simulink model "Hinf_design"  (R2019b)
settings: Solver=ode14x  StartTime=0.0  StopTime=experiment.stop_time  FixedStep=0.002  RelTol=1e-3
values from neighbouring files (symbols this model uses):
  B_1 = B    (= 0.0015)    [nominal_model.m]
  B_2 = B    (= 0.0015)    [nominal_model.m]
  B_eq = 0.015    [nominal_model.m]
  data = e_h.load_data    [potentiometer_recover.m]
  eta_g = 0.9    [nominal_model.m]
  eta_m = 0.69    [nominal_model.m]
  experiment = merge( experiment, experiment2 )    [blackbox_est.m]
  J_1 = J    (= 0.000545)    [nominal_model.m]
  J_2 = J    (= 0.000545)    [nominal_model.m]
  J_eq = 2.087e-3    (= 0.002087)    [nominal_model.m]
  K_g = 70    [nominal_model.m]
  k_m = 7.68e-3    (= 0.00768)    [nominal_model.m]
  K_s1 = K_s    (= 1)    [nominal_model.m]
  K_s2 = K_s    (= 1)    [nominal_model.m]
  k_t = 7.68e-3    (= 0.00768)    [nominal_model.m]
  Lm = 0.18e-3    (= 0.00018)    [nominal_model.m]
  Rm = 2.6    [nominal_model.m]
  V_max = 10    [nominal_model.m]
undefined symbols (not defined in the file or in its folder): active_dof, controller, encoder_var, potentiometer_var
libraries: simulink x12
settings Model: Creator=giacomo  LastModifiedBy=denniszanutto

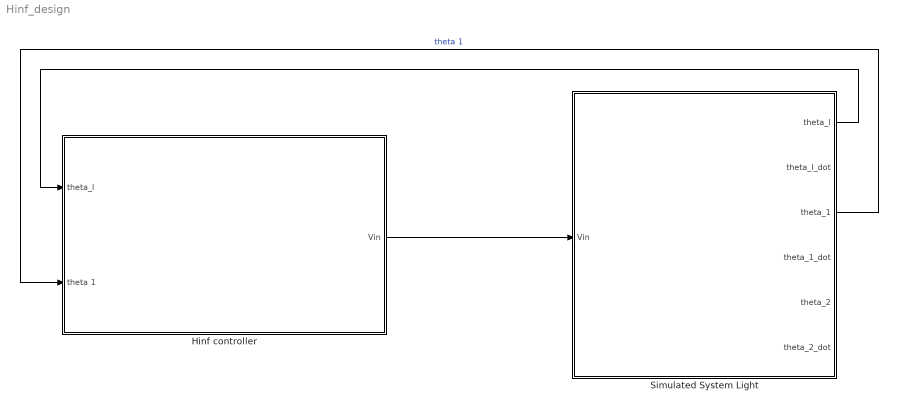
== system Hinf_design ==
  Hinf controller : Subsystem
  Simulated System Light : Subsystem
  wires:
  Simulated System Light/1(theta_l) -> Hinf controller/1(theta_l)
  Simulated System Light/3(theta_1) -> Hinf controller/2(theta 1)  "theta 1"
  Hinf controller/1(Vin) -> Simulated System Light/1(Vin)

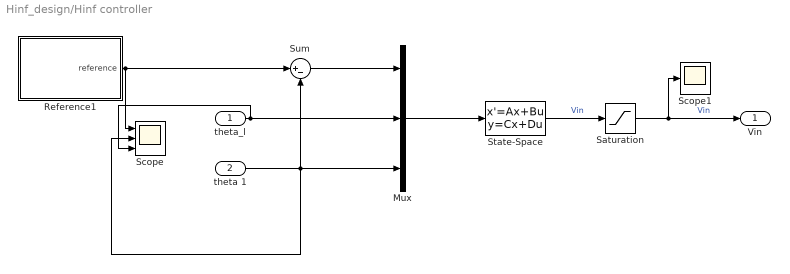
== system Hinf_design/Hinf controller ==
  theta_l : Inport
  theta 1 : Inport  Port=2
  Mux : Mux  Inputs=3
  Reference1 : Subsystem
  Saturation : Saturate  UpperLimit=V_max  LowerLimit=-V_max
  Scope : Scope  NumInputPorts=3
  Scope1 : Scope
  State-Space : StateSpace  A=controller.c11.A  B=controller.c11.B  C=controller.c11.C  D=controller.c11.D  InitialCondition=0
  Sum : Sum  Inputs=|+-
  Vin : Outport
  wires:
  Reference1/1(reference) -> Sum/1, Scope/1
  State-Space/1 -> Saturation/1  "Vin"
  Sum/1 -> Mux/1
  theta_l/1 -> Scope/3, Mux/2
  theta 1/1 -> Scope/2, Mux/3, Sum/2
  Mux/1 -> State-Space/1
  Saturation/1 -> Vin/1, Scope1/1  "Vin"

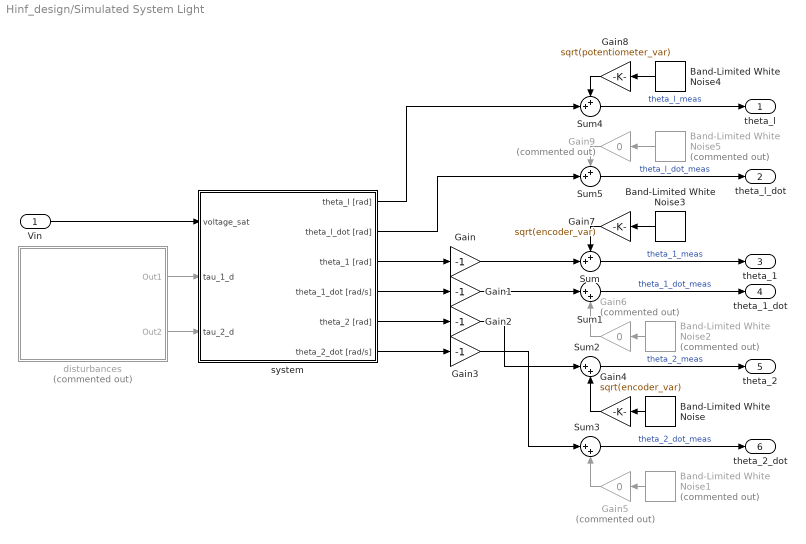
== system Hinf_design/Simulated System Light ==
  Vin : Inport
  Band-Limited White Noise : simulink/Sources/Band-Limited White Noise  Cov=1  Ts=0.002  seed=[23341]
  Band-Limited White Noise1 : simulink/Sources/Band-Limited White Noise  Commented=on  Cov=1  Ts=0.002  seed=[23341]
  Band-Limited White Noise2 : simulink/Sources/Band-Limited White Noise  Commented=on  Cov=1  Ts=0.002  seed=[23341]
  Band-Limited White Noise3 : simulink/Sources/Band-Limited White Noise  Cov=1  Ts=0.002  seed=[23341]
  Band-Limited White Noise4 : simulink/Sources/Band-Limited White Noise  Cov=1  Ts=0.002  seed=[23341]
  Band-Limited White Noise5 : simulink/Sources/Band-Limited White Noise  Commented=on  Cov=1  Ts=0.002  seed=[23341]
  Gain{,1..3} (4 alike) : Gain  Gain=-1
  Gain4 : Gain  Gain=sqrt(encoder_var)
  Gain5 : Gain  Commented=on  Gain=0
  Gain6 : Gain  Commented=on  Gain=0
  Gain7 : Gain  Gain=sqrt(encoder_var)
  Gain8 : Gain  Gain=sqrt(potentiometer_var)
  Gain9 : Gain  Commented=on  Gain=0
  Sum : Sum  Inputs=++|
  Sum1 : Sum  Inputs=|++
  Sum2 : Sum  Inputs=|++
  Sum3 : Sum  Inputs=|++
  Sum4 : Sum  Inputs=++|
  Sum5 : Sum  Inputs=++|
  disturbances : Subsystem  Commented=on
  system : Subsystem
  theta_l : Outport
  theta_l_dot : Outport  Port=2
  theta_1 : Outport  Port=3
  theta_1_dot : Outport  Port=4
  theta_2 : Outport  Port=5
  theta_2_dot : Outport  Port=6
  wires:
  system/5(theta_2 [rad]) -> Gain2/1
  system/6(theta_2_dot [rad/s]) -> Gain3/1
  system/4(theta_1_dot [rad/s]) -> Gain1/1
  Vin/1 -> system/1(voltage_sat)
  Gain/1 -> Sum/2
  Gain2/1 -> Sum2/1
  system/3(theta_1 [rad]) -> Gain/1
  Sum/1 -> theta_1/1  "theta_1_meas"
  Sum1/1 -> theta_1_dot/1  "theta_1_dot_meas"
  Sum2/1 -> theta_2/1  "theta_2_meas"
  Gain3/1 -> Sum3/1
  Sum3/1 -> theta_2_dot/1  "theta_2_dot_meas"
  Gain4/1 -> Sum2/2
  Band-Limited White Noise/1 -> Gain4/1
  Band-Limited White Noise1/1 -> Gain5/1
  Gain5/1 -> Sum3/2
  Band-Limited White Noise2/1 -> Gain6/1
  Gain7/1 -> Sum/1
  Band-Limited White Noise3/1 -> Gain7/1
  Gain8/1 -> Sum4/1
  Band-Limited White Noise4/1 -> Gain8/1
  Sum4/1 -> theta_l/1  "theta_l_meas"
  Sum5/1 -> theta_l_dot/1  "theta_l_dot_meas"
  Band-Limited White Noise5/1 -> Gain9/1
  Gain9/1 -> Sum5/1
  system/2(theta_l_dot [rad]) -> Sum5/2
  system/1(theta_l [rad]) -> Sum4/2
  Gain1/1 -> Sum1/1
  Gain6/1 -> Sum1/2
  disturbances/1(Out1) -> system/2(tau_1_d)
  disturbances/2(Out2) -> system/3(tau_2_d)

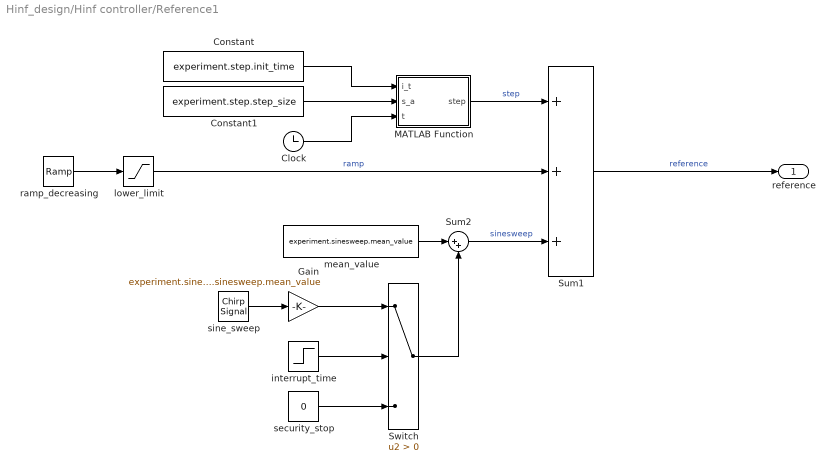
== system Hinf_design/Hinf controller/Reference1 ==
  Clock : Clock
  Constant : Constant  Value=experiment.step.init_time
  Constant1 : Constant  Value=experiment.step.step_size
  Gain : Gain  Gain=experiment.sinesweep.v_max-experiment.sinesweep.mean_value
  MATLAB Function : MATLAB Function  TreatAsAtomicUnit=on
  Sum1 : Sum  Inputs=+++
  Sum2 : Sum  Inputs=|++
  Switch : Switch  Criteria=u2 > Threshold
  interrupt_time : Step  Time=experiment.sinesweep.target_time  Before=1  After=-1  SampleTime=0
  lower_limit : Saturate  UpperLimit=max( experiment.ramp.init_value, experiment.ramp.final_value )  LowerLimit=min( experiment.ramp.init_value, experiment.ramp.final_value )
  mean_value : Constant  Value=experiment.sinesweep.mean_value
  ramp_decreasing : simulink/Sources/Ramp  slope=experiment.ramp.ramp_pend  start=experiment.ramp.init_time  InitialOutput=experiment.ramp.init_value
  security_stop : Constant  Value=0
  sine_sweep : simulink/Sources/Chirp Signal  f1=experiment.sinesweep.init_freq  T=experiment.sinesweep.target_time  f2=experiment.sinesweep.final_freq
  reference : Outport
  wires:
  mean_value/1 -> Sum2/1
  lower_limit/1 -> Sum1/2  "ramp"
  Switch/1 -> Sum2/2
  interrupt_time/1 -> Switch/2
  Sum2/1 -> Sum1/3  "sinesweep"
  Sum1/1 -> reference/1  "reference"
  security_stop/1 -> Switch/3
  ramp_decreasing/1 -> lower_limit/1
  Gain/1 -> Switch/1
  sine_sweep/1 -> Gain/1
  Clock/1 -> MATLAB Function/3(t)
  Constant/1 -> MATLAB Function/1(i_t)
  Constant1/1 -> MATLAB Function/2(s_a)
  MATLAB Function/1(step) -> Sum1/1  "step"

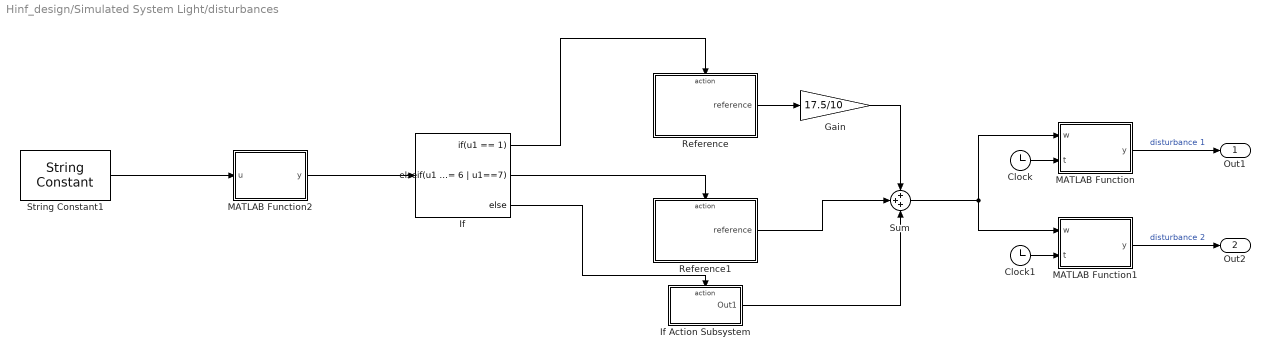
== system Hinf_design/Simulated System Light/disturbances ==
  Clock : Clock
  Clock1 : Clock
  Gain : Gain  Gain=17.5/10
  If : If  IfExpression=u1 == 1  ElseIfExpressions=u1 == 5 | u1 == 6 | u1==7
  If Action Subsystem : Subsystem  TreatAsAtomicUnit=on
  MATLAB Function : MATLAB Function  TreatAsAtomicUnit=on
  MATLAB Function1 : MATLAB Function  TreatAsAtomicUnit=on
  MATLAB Function2 : MATLAB Function  TreatAsAtomicUnit=on
  Reference : Subsystem
  Reference1 : Subsystem
  String Constant1 : StringConstant  String=experiment.refVariable
  Sum : Sum  Inputs=+++
  Out1 : Outport
  Out2 : Outport  Port=2
  wires:
  Clock/1 -> MATLAB Function/2(t)
  MATLAB Function/1(y) -> Out1/1  "disturbance 1"
  Clock1/1 -> MATLAB Function1/2(t)
  MATLAB Function1/1(y) -> Out2/1  "disturbance 2"
  Reference/1(reference) -> Gain/1
  If/1 -> Reference/Action
  MATLAB Function2/1(y) -> If/1
  If/2 -> Reference1/Action
  If/3 -> If Action Subsystem/Action
  Gain/1 -> Sum/1
  Reference1/1(reference) -> Sum/2
  If Action Subsystem/1(Out1) -> Sum/3
  Sum/1 -> MATLAB Function1/1(w), MATLAB Function/1(w)
  String Constant1/1 -> MATLAB Function2/1(u)

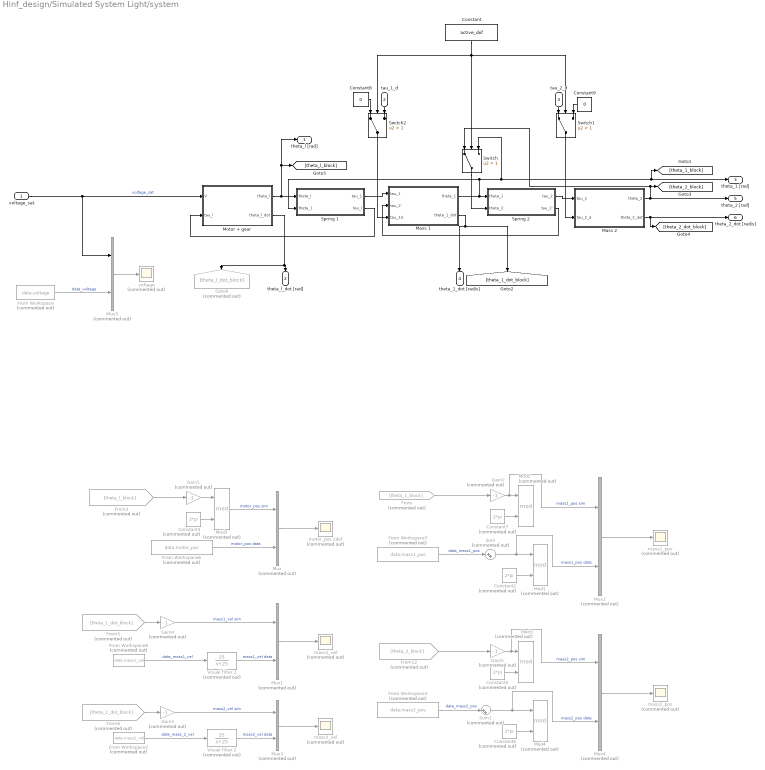
== system Hinf_design/Simulated System Light/system ==
  voltage_sat : Inport
  tau_1_d : Inport  Port=2
  tau_2_d : Inport  Port=3
  Constant : Constant  Value=active_dof
  Constant{2..4,6..7} (5 alike) : Constant  Commented=on  Value=2*pi
  Constant8 : Constant  Value=0
  Constant9 : Constant  Value=0
  From : From  Commented=on  GotoTag=theta_1_block
  From Workspace : FromWorkspace  Commented=on  VariableName=data.voltage  SampleTime=0
  From Workspace2 : FromWorkspace  Commented=on  VariableName=data.mass2_vel  SampleTime=0.002
  From Workspace3 : FromWorkspace  Commented=on  VariableName=data.mass2_pos  SampleTime=0.002
  From Workspace6 : FromWorkspace  Commented=on  VariableName=data.motor_pos  SampleTime=0.002
  From Workspace7 : FromWorkspace  Commented=on  VariableName=data.mass1_pos  SampleTime=0.002
  From Workspace8 : FromWorkspace  Commented=on  VariableName=data.mass1_vel  SampleTime=0.002
  From12 : From  Commented=on  GotoTag=theta_2_block
  From3 : From  Commented=on  GotoTag=theta_l_block
  From5 : From  Commented=on  GotoTag=theta_1_dot_block
  From6 : From  Commented=on  GotoTag=theta_2_dot_block
  Gain{1..5} (5 alike) : Gain  Commented=on  Gain=-1
  Goto6 : Goto  Commented=on  GotoTag=theta_l_dot_block
  Mass 1 : Subsystem
  Mass 2 : Subsystem
  Mod{1..5} (5 alike) : Math  Commented=on  Operator=mod  SignedPower=off  SaturateOnIntegerOverflow=on
  Motor + gear : Subsystem
  Mux{,1..5} (6 alike) : Mux  Commented=on  Inputs=2
  Spring 1 : Subsystem
  Spring 2 : Subsystem
  Sum : Sum  Commented=on  Inputs=|++
  Sum1 : Sum  Commented=on  Inputs=|++
  Switch : Switch  Criteria=u2 > Threshold  Threshold=1
  Switch1 : Switch  Criteria=u2 > Threshold  Threshold=1
  Switch2 : Switch  Criteria=u2 > Threshold  Threshold=1
  Visual filter 1 : TransferFcn  Commented=on  Numerator=[25]  Denominator=[1 25]
  Visual filter 2 : TransferFcn  Commented=on  Numerator=[25]  Denominator=[1 25]
  mass1_pos : Scope  Commented=on
  mass1_vel : Scope  Commented=on
  mass2_pos : Scope  Commented=on
  mass2_vel : Scope  Commented=on
  motor_pos 2dof : Scope  Commented=on
  voltage : Scope  Commented=on
  theta_l [rad] : Outport
  theta_l_dot [rad] : Outport  Port=2
  theta_1 [rad] : Outport  Port=3
  theta_1_dot [rad/s] : Outport  Port=4
  theta_2 [rad] : Outport  Port=5
  theta_2_dot [rad/s] : Outport  Port=6
  wires:
  Spring 1/1(tau_1) -> Mass 1/1(tau_1)
  voltage_sat/1 -> Motor + gear/1(V), Mux5/1  "voltage_sat"
  Spring 1/2(tau_l) -> Motor + gear/2(tau_l)
  Spring 2/2(tau_2') -> Mass 1/2(tau_2')
  Spring 2/1(tau_2) -> Mass 2/1(tau_2)
  From Workspace6/1 -> Mux/2  "motor_pos data"
  Visual filter 1/1 -> Mux1/2  "mass1_vel data"
  From Workspace7/1 -> Sum/1  "data_mass1_pos"
  Sum/1 -> Mux2/2, Mod1/1  "mass1_pos data"
  Constant2/1 -> Mod1/2
  From5/1 -> Gain4/1
  Mux/1 -> motor_pos 2dof/1
  Mux1/1 -> mass1_vel/1
  From Workspace8/1 -> Visual filter 1/1  "data_mass1_vel"
  Mux2/1 -> mass1_pos/1
  From Workspace2/1 -> Visual filter 2/1  "data_mass_2_vel"
  Mux3/1 -> mass2_vel/1
  Visual filter 2/1 -> Mux3/2  "mass2_vel data"
  From6/1 -> Gain3/1
  Mux4/1 -> mass2_pos/1
  From Workspace3/1 -> Sum1/1  "data_mass2_pos"
  Sum1/1 -> Mux4/2, Mod4/1  "mass2_pos data"
  Constant6/1 -> Mod4/2
  From12/1 -> Gain5/1
  Motor + gear/1(theta_l) -> theta_l [rad]/1, [theta_l_block], Spring 1/1(theta_l)
  Mass 1/2(theta_1_dot) -> [theta_1_dot_block], theta_1_dot [rad/s]/1
  Mass 2/1(theta_2) -> [theta_2_block], Switch/1, theta_2 [rad]/1
  Mass 2/2(theta_2_dot) -> [theta_2_dot_block], theta_2_dot [rad/s]/1
  Switch/1 -> Spring 2/2(theta_2)
  Mass 1/1(theta_1) -> Switch/3, [theta_1_block], theta_1 [rad]/1, Spring 1/2(theta_1), Spring 2/1(theta_1)
  Switch1/1 -> Mass 2/2(tau_2_d)
  tau_2_d/1 -> Switch1/1
  Constant9/1 -> Switch1/3
  Constant/1 -> Switch/2, Switch2/2, Switch1/2
  Constant8/1 -> Switch2/1
  tau_1_d/1 -> Switch2/3
  Switch2/1 -> Mass 1/3(tau_1d)
  Gain3/1 -> Mux3/1  "mass2_vel sim"
  Gain4/1 -> Mux1/1  "mass1_vel sim"
  Gain2/1 -> Mux2/1, Mod5/1  "mass1_pos sim"
  Constant7/1 -> Mod5/2
  From/1 -> Gain2/1
  Constant3/1 -> Mod2/2
  Gain1/1 -> Mod2/1
  Mod2/1 -> Mux/1  "motor_pos sim"
  From3/1 -> Gain1/1
  Gain5/1 -> Mux4/1, Mod3/1  "mass2_pos sim"
  Constant4/1 -> Mod3/2
  Motor + gear/2(theta_l_dot) -> theta_l_dot [rad]/1, Goto6/1
  From Workspace/1 -> Mux5/2  "data_voltage"
  Mux5/1 -> voltage/1

== system Hinf_design/Simulated System Light/disturbances/If Action Subsystem ==
  Action Port : ActionPort  ActionPortLabel=else
  Constant : Constant  Value=0
  Out1 : Outport
  wires:
  Constant/1 -> Out1/1

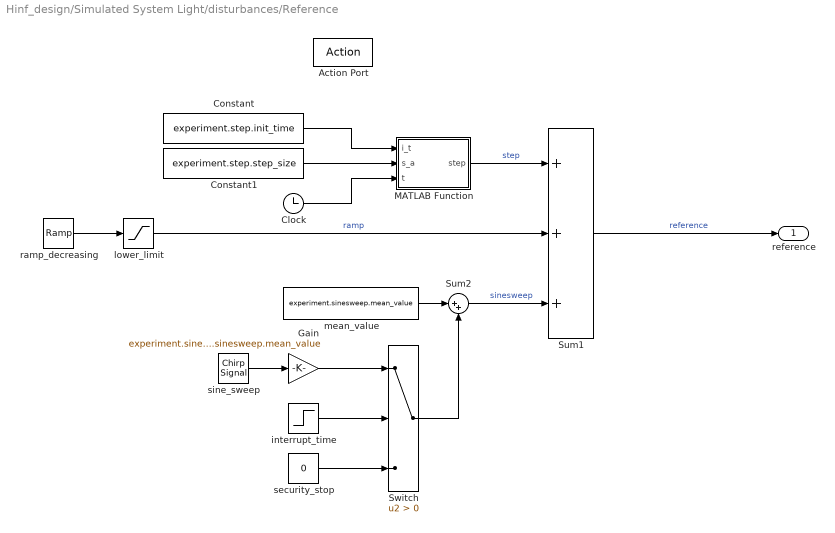
== system Hinf_design/Simulated System Light/disturbances/Reference ==
  Action Port : ActionPort  ActionPortLabel=if(u1 == 1)
  Clock : Clock
  Constant : Constant  Value=experiment.step.init_time
  Constant1 : Constant  Value=experiment.step.step_size
  Gain : Gain  Gain=experiment.sinesweep.v_max-experiment.sinesweep.mean_value
  MATLAB Function : MATLAB Function  TreatAsAtomicUnit=on
  Sum1 : Sum  Inputs=+++
  Sum2 : Sum  Inputs=|++
  Switch : Switch  Criteria=u2 > Threshold
  interrupt_time : Step  Time=experiment.sinesweep.target_time  Before=1  After=-1  SampleTime=0
  lower_limit : Saturate  UpperLimit=max( experiment.ramp.init_value, experiment.ramp.final_value )  LowerLimit=min( experiment.ramp.init_value, experiment.ramp.final_value )
  mean_value : Constant  Value=experiment.sinesweep.mean_value
  ramp_decreasing : simulink/Sources/Ramp  slope=experiment.ramp.ramp_pend  start=experiment.ramp.init_time  InitialOutput=experiment.ramp.init_value
  security_stop : Constant  Value=0
  sine_sweep : simulink/Sources/Chirp Signal  f1=experiment.sinesweep.init_freq  T=experiment.sinesweep.target_time  f2=experiment.sinesweep.final_freq
  reference : Outport
  wires:
  mean_value/1 -> Sum2/1
  lower_limit/1 -> Sum1/2  "ramp"
  Switch/1 -> Sum2/2
  interrupt_time/1 -> Switch/2
  Sum2/1 -> Sum1/3  "sinesweep"
  Sum1/1 -> reference/1  "reference"
  security_stop/1 -> Switch/3
  ramp_decreasing/1 -> lower_limit/1
  Gain/1 -> Switch/1
  sine_sweep/1 -> Gain/1
  Clock/1 -> MATLAB Function/3(t)
  Constant/1 -> MATLAB Function/1(i_t)
  Constant1/1 -> MATLAB Function/2(s_a)
  MATLAB Function/1(step) -> Sum1/1  "step"

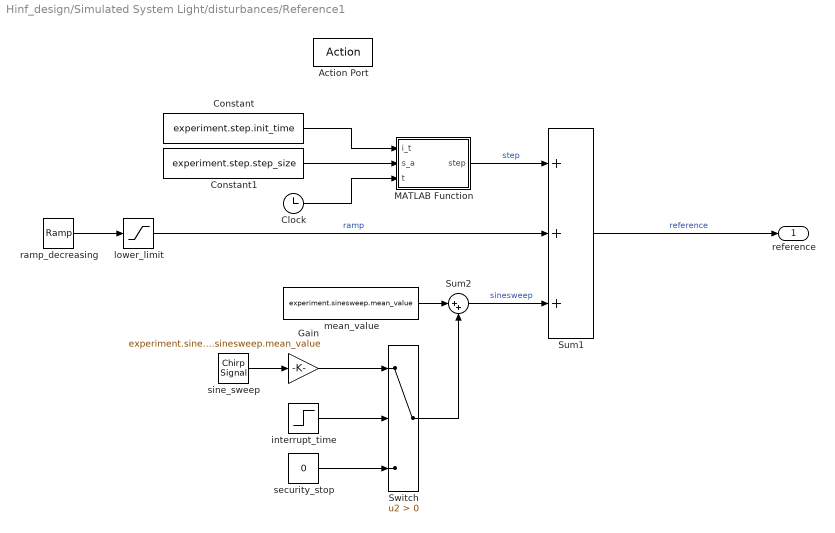
== system Hinf_design/Simulated System Light/disturbances/Reference1 ==
  Action Port : ActionPort  ActionPortLabel=elseif(u1 == 5 | u1 == 6 | u1==7)
  Clock : Clock
  Constant : Constant  Value=experiment.step.init_time
  Constant1 : Constant  Value=experiment.step.step_size
  Gain : Gain  Gain=experiment.sinesweep.v_max-experiment.sinesweep.mean_value
  MATLAB Function : MATLAB Function  TreatAsAtomicUnit=on
  Sum1 : Sum  Inputs=+++
  Sum2 : Sum  Inputs=|++
  Switch : Switch  Criteria=u2 > Threshold
  interrupt_time : Step  Time=experiment.sinesweep.target_time  Before=1  After=-1  SampleTime=0
  lower_limit : Saturate  UpperLimit=max( experiment.ramp.init_value, experiment.ramp.final_value )  LowerLimit=min( experiment.ramp.init_value, experiment.ramp.final_value )
  mean_value : Constant  Value=experiment.sinesweep.mean_value
  ramp_decreasing : simulink/Sources/Ramp  slope=experiment.ramp.ramp_pend  start=experiment.ramp.init_time  InitialOutput=experiment.ramp.init_value
  security_stop : Constant  Value=0
  sine_sweep : simulink/Sources/Chirp Signal  f1=experiment.sinesweep.init_freq  T=experiment.sinesweep.target_time  f2=experiment.sinesweep.final_freq
  reference : Outport
  wires:
  mean_value/1 -> Sum2/1
  lower_limit/1 -> Sum1/2  "ramp"
  Switch/1 -> Sum2/2
  interrupt_time/1 -> Switch/2
  Sum2/1 -> Sum1/3  "sinesweep"
  Sum1/1 -> reference/1  "reference"
  security_stop/1 -> Switch/3
  ramp_decreasing/1 -> lower_limit/1
  Gain/1 -> Switch/1
  sine_sweep/1 -> Gain/1
  Clock/1 -> MATLAB Function/3(t)
  Constant/1 -> MATLAB Function/1(i_t)
  Constant1/1 -> MATLAB Function/2(s_a)
  MATLAB Function/1(step) -> Sum1/1  "step"

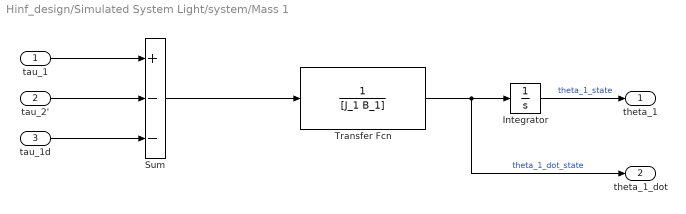
== system Hinf_design/Simulated System Light/system/Mass 1 ==
  tau_1 : Inport
  tau_2' : Inport  Port=2
  tau_1d : Inport  Port=3
  Integrator : Integrator  InitialCondition=data.motor_pos_0
  Sum : Sum  Inputs=+--
  Transfer Fcn : TransferFcn  Denominator=[J_1 B_1]
  theta_1 : Outport
  theta_1_dot : Outport  Port=2
  wires:
  tau_1/1 -> Sum/1
  tau_2'/1 -> Sum/2
  Sum/1 -> Transfer Fcn/1
  Transfer Fcn/1 -> theta_1_dot/1, Integrator/1  "theta_1_dot_state"
  Integrator/1 -> theta_1/1  "theta_1_state"
  tau_1d/1 -> Sum/3

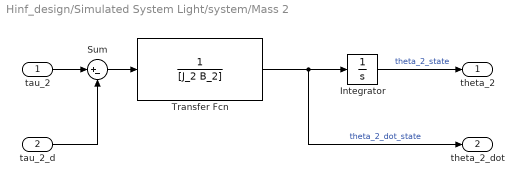
== system Hinf_design/Simulated System Light/system/Mass 2 ==
  tau_2 : Inport
  tau_2_d : Inport  Port=2
  Integrator : Integrator  InitialCondition=data.motor_pos_0
  Sum : Sum  Inputs=|+-
  Transfer Fcn : TransferFcn  Denominator=[J_2 B_2]
  theta_2 : Outport
  theta_2_dot : Outport  Port=2
  wires:
  Transfer Fcn/1 -> theta_2_dot/1, Integrator/1  "theta_2_dot_state"
  Integrator/1 -> theta_2/1  "theta_2_state"
  tau_2/1 -> Sum/1
  Sum/1 -> Transfer Fcn/1
  tau_2_d/1 -> Sum/2

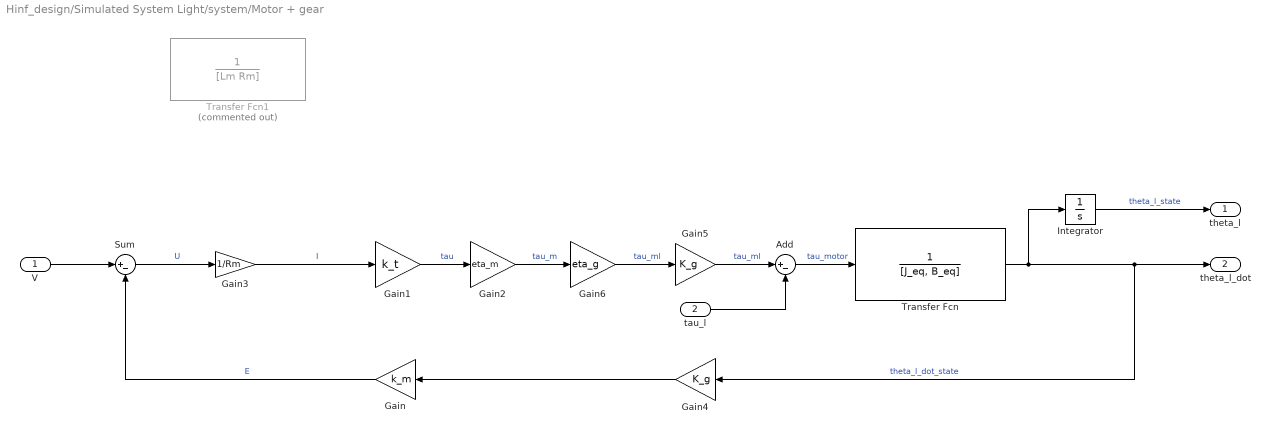
== system Hinf_design/Simulated System Light/system/Motor + gear ==
  V : Inport
  tau_l : Inport  Port=2
  Add : Sum  Inputs=|+-
  Gain : Gain  Gain=k_m
  Gain1 : Gain  Gain=k_t
  Gain2 : Gain  Gain=eta_m
  Gain3 : Gain  Gain=1/Rm
  Gain4 : Gain  Gain=K_g
  Gain5 : Gain  Gain=K_g
  Gain6 : Gain  Gain=eta_g
  Integrator : Integrator  InitialCondition=data.motor_pos_0
  Sum : Sum  Inputs=|+-
  Transfer Fcn : TransferFcn  Denominator=[J_eq, B_eq]
  Transfer Fcn1 : TransferFcn  Commented=on  Denominator=[Lm Rm]
  theta_l : Outport
  theta_l_dot : Outport  Port=2
  wires:
  V/1 -> Sum/1
  Sum/1 -> Gain3/1  "U"
  Gain/1 -> Sum/2  "E"
  Gain3/1 -> Gain1/1  "I"
  Gain1/1 -> Gain2/1  "tau"
  Gain6/1 -> Gain5/1  "tau_ml"
  Transfer Fcn/1 -> Gain4/1, theta_l_dot/1, Integrator/1  "theta_l_dot_state"
  Gain4/1 -> Gain/1
  tau_l/1 -> Add/2
  Gain5/1 -> Add/1  "tau_ml"
  Gain2/1 -> Gain6/1  "tau_m"
  Integrator/1 -> theta_l/1  "theta_l_state"
  Add/1 -> Transfer Fcn/1  "tau_motor"

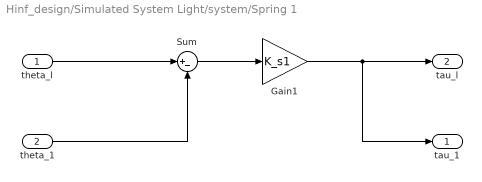
== system Hinf_design/Simulated System Light/system/Spring 1 ==
  theta_l : Inport
  theta_1 : Inport  Port=2
  Gain1 : Gain  Gain=K_s1
  Sum : Sum  Inputs=|+-
  tau_1 : Outport
  tau_l : Outport  Port=2
  wires:
  Sum/1 -> Gain1/1
  Gain1/1 -> tau_1/1, tau_l/1
  theta_l/1 -> Sum/1
  theta_1/1 -> Sum/2

== system Hinf_design/Simulated System Light/system/Spring 2 ==
  theta_1 : Inport
  theta_2 : Inport  Port=2
  Gain1 : Gain  Gain=K_s2
  Sum : Sum  Inputs=|+-
  tau_2 : Outport
  tau_2' : Outport  Port=2
  wires:
  Sum/1 -> Gain1/1
  Gain1/1 -> tau_2'/1, tau_2/1
  theta_1/1 -> Sum/1
  theta_2/1 -> Sum/2

== matlab function Hinf_design/Hinf controller/Reference1/MATLAB Function ==
  data: i_t input; step output; s_a input; t input
function step = multistep(i_t, s_a, t)

% it is assumed i_t is sorted!

% find the first time step that is greater than actual time. 
step = 0;
for idx = 1:length(i_t) 
    if i_t(idx) <= t
        step = s_a(idx);
    end
end

== matlab function Hinf_design/Simulated System Light/disturbances/MATLAB Function ==
  data: w input; y output; t input
function y = fcn(w,t)
    if abs(w) < 1
        A = 0.001;
    else
        A = 0.005;
    end
y = A*sin(w*t);

== matlab function Hinf_design/Simulated System Light/disturbances/MATLAB Function1 ==
  data: w input; y output; t input
function y = fcn(w,t)
    if abs(w) < 1
        A = 0;
    else
        A = 0.005;
    end
y = A*sin(w*t);

== matlab function Hinf_design/Simulated System Light/disturbances/Reference/MATLAB Function ==
  data: i_t input; step output; s_a input; t input
function step = multistep(i_t, s_a, t)

% it is assumed i_t is sorted!

% find the first time step that is greater than actual time. 
step = 0;
for idx = 1:length(i_t) 
    if i_t(idx) <= t
        step = s_a(idx);
    end
end

== matlab function Hinf_design/Simulated System Light/disturbances/Reference1/MATLAB Function ==
  data: i_t input; step output; s_a input; t input
function step = multistep(i_t, s_a, t)

% it is assumed i_t is sorted!

% find the first time step that is greater than actual time. 
step = 0;
for idx = 1:length(i_t) 
    if i_t(idx) <= t
        step = s_a(idx);
    end
end

== matlab function Hinf_design/Simulated System Light/disturbances/MATLAB Function2 ==
  data: u input; y output
function y = fcn(u)
if strcmp( u, 'voltage')
    y = 1;
elseif strcmp( u, 'motor_pos')
    y = 2;
elseif strcmp( u, 'mass1_pos' )
    y = 3;
elseif strcmp( u, 'mass2_pos')
    y = 4;
elseif strcmp( u, 'motor_vel' )
    y = 5;
elseif strcmp( u, 'mass1_vel')
    y = 6;
else 
    y = 7;
end
end
